simulink model "sl_subsys_fcncallerr3"  (Simulink 7.6)
settings: Solver=FixedStepDiscrete  StartTime=0.0  StopTime=10.0  FixedStep=1  RelTol=1e-3
Description:
  | Data dependency violation involving block between two function-call subsystems
  | 
  | The following model is an illegal example of a chart that executes a function-call
  | subsystem that in turn executes another function-call subsystem. The Chart is making
  | the function-call [d1,d2]=f(),, i.e., invoking f() and then later using the values
  | d1 and d2. As defined by the diagram, f() is attempting to make the call
  | g(B(out2)). However, the block B is not contained within f() and thus cannot
  | be executed when expected, resulting in a data dependency violation.
settings Model: Creator=The MathWorks Inc.  CovMetricSettings=d  ExtModeAutoUpdateStatusClock=off
settings OptimizationCC: BlockReduction=off  BooleanDataType=off  InlineInvariantSignals=on  InitFltsAndDblsToZero=on
settings DebuggingCC: SaveWithParameterizedLinksMsg=none  SignalResolutionControl=TryResolveAllWithWarning  SolverPrmCheckMsg=none  MultiTaskDSMMsg=warning  MultiTaskCondExecSysMsg=none
settings HardwareCC: TargetUnknown=on
settings SFSimCC: SimParseCustomCode=off
settings RTWCC: IncludeERTFirstTime=on
settings CodeAppCC: CustomSymbolStrFcn=$F$N$M
settings GRTTargetCC: TargetFcnLib=ansi_tfl_tmw.mat

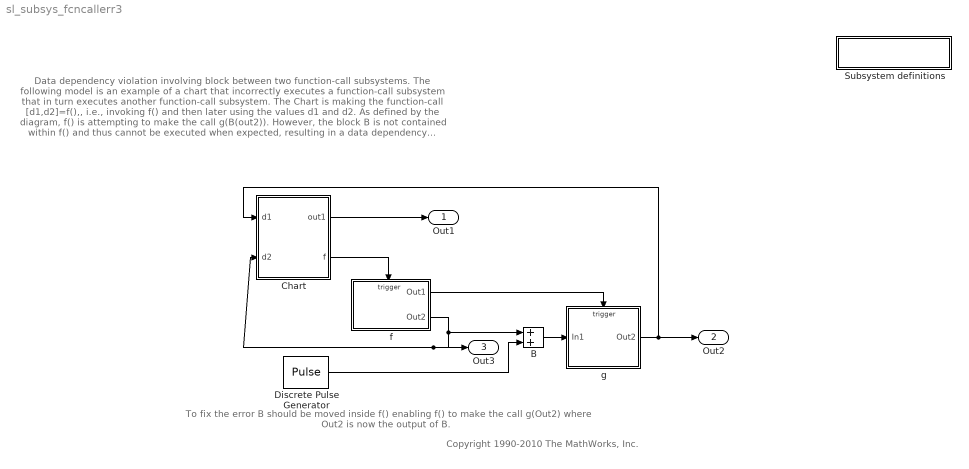
== system sl_subsys_fcncallerr3 ==
  note: Data dependency violation involving block between two function-call subsystems.
      |
      | The following model is an example of a chart that incorrectly executes a function-call
      | subsystem that in turn executes another function-call subsystem. The Chart is making
      | the function-call [d1,d2]=f(),, i.e., invoking f() and then later using the values
      | d1 and d2. As defined by the diagram, f() is attempting to make the call
      | g(B(out2)). However, the block B is not contained within f() and thus cannot
      | be executed when expected, resulting in a data dependency violation.
  note: To fix the error B should be moved inside f() enabling f()
      | to make the call g(Out2) where Out2 is now the output of B.
  note: Copyright 1990-2010 The MathWorks, Inc.
  " Subsystem definitions" : Subsystem
      settings: OpenFcn=helpview([matlabroot,'/toolbox/simulink/simdemos/simfeatures/html/sl_subsys_definitions.html']);
      mask Display: disp('Subsystem\ndefinitions')
  B : Sum  SaturateOnIntegerOverflow=on  InputSameDT=on  OutDataTypeStr=Inherit: Same as first input
  Chart : Stateflow chart  TreatAsAtomicUnit=on
  Discrete Pulse Generator : DiscretePulseGenerator
  f : Subsystem  TreatAsAtomicUnit=on
  g : Subsystem  TreatAsAtomicUnit=on
  Out1 : Outport
  Out2 : Outport  Port=2
  Out3 : Outport  Port=3
  wires:
  Chart/2(f) -> f/Trigger
  f/1(Out1) -> g/Trigger
  f/2(Out2) -> Out3/1, Chart/2(d2), B/1
  g/1(Out2) -> Out2/1, Chart/1(d1)
  Chart/1(out1) -> Out1/1
  Discrete Pulse Generator/1 -> B/2
  B/1 -> g/1(In1)

== system sl_subsys_fcncallerr3/ Subsystem definitions ==

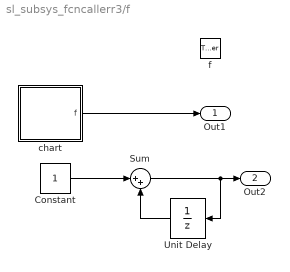
== system sl_subsys_fcncallerr3/f ==
  f : TriggerPort  TriggerType=function-call
  Constant : Constant
  Sum : Sum  Inputs=|++  SaturateOnIntegerOverflow=on  InputSameDT=on  OutDataTypeStr=Inherit: Same as first input
  Unit Delay : UnitDelay  SampleTime=-1
  chart : Stateflow chart  TreatAsAtomicUnit=on
  Out1 : Outport
  Out2 : Outport  Port=2
  wires:
  chart/1(f) -> Out1/1
  Constant/1 -> Sum/1
  Unit Delay/1 -> Sum/2
  Sum/1 -> Out2/1, Unit Delay/1

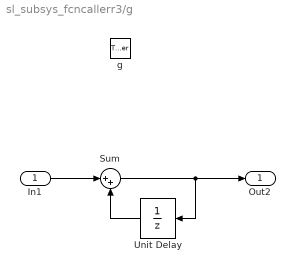
== system sl_subsys_fcncallerr3/g ==
  In1 : Inport
  g : TriggerPort  TriggerType=function-call
  Sum : Sum  Inputs=|++  SaturateOnIntegerOverflow=on  InputSameDT=on  OutDataTypeStr=Inherit: Same as first input
  Unit Delay : UnitDelay  SampleTime=-1
  Out2 : Outport
  wires:
  In1/1 -> Sum/1
  Unit Delay/1 -> Sum/2
  Sum/1 -> Out2/1, Unit Delay/1

== stateflow chart Chart ==
  state one/
    entry:f;out1=d1+d2;
  state two/
    entry: f;out1=d1-d2;
  one -> two
  two -> one
  (default) -> one
  data: d1 input double; d2 input double; out1 output double; out local double
  events: f output FUNCTION_CALL_EVENT

== stateflow chart f/chart ==
  state one/
    entry: f;
  state two/
    entry: f;
  one -> two
  two -> one
  (default) -> one
  events: f output FUNCTION_CALL_EVENT
